simulink model "REV3"  (R2025b)
settings: Solver=ode8  StartTime=0.0  StopTime=inf  FixedStep=0.0001  RelTol=1e-3
undefined symbols (not defined in the file): BMS_Contactor_Command, MC_DC_State, MC_VSM_State, UC_State
(part 2 of 2)

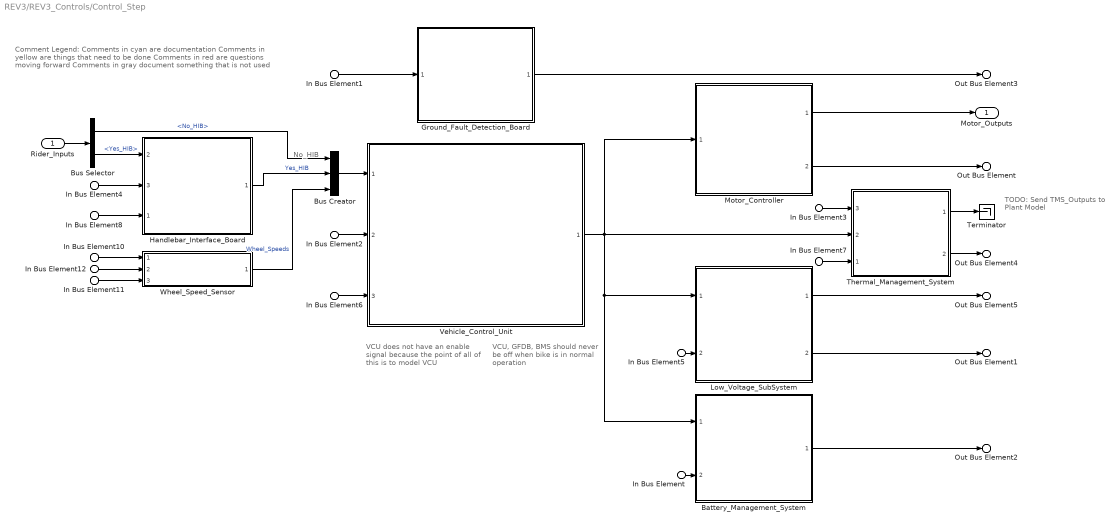
== system REV3/REV3_Controls/Control_Step ==
  note: VCU does not have an enable signal because the point of all of this is to model VCU
  note: No_HIB
  note: TODO: Send TMS_Outputs to Plant Model
  note: VCU, GFDB, BMS should never be off when bike is in normal operation
  note: Comment Legend:
      | Comments in cyan are documentation
      | Comments in yellow are things that need to be done
      | Comments in red are questions moving forward
      | Comments in gray document something that is not used
  Rider_Inputs : Inport
  In Bus Element2 : Inport  Port=2  PortName=Fault_Inputs  Element=VCU
  In Bus Element3 : Inport  Port=2  PortName=Fault_Inputs  Element=TMS
  In Bus Element4 : Inport  Port=2  PortName=Fault_Inputs  Element=HIB
  In Bus Element5 : Inport  Port=2  PortName=Fault_Inputs  Element=LVSS
  In Bus Element : Inport  Port=2  PortName=Fault_Inputs  Element=BMS
  In Bus Element1 : Inport  Port=2  PortName=Fault_Inputs  Element=GFDB
  In Bus Element12 : Inport  Port=2  PortName=Fault_Inputs  Element=WSS
  In Bus Element11 : Inport  Port=3  PortName=Sensor_Inputs
  In Bus Element6 : Inport  Port=4  PortName=Feedback_Input
  In Bus Element8 : Inport  Port=4  PortName=Feedback_Input  Element=LVSS_Outputs.HIB_Power
  In Bus Element7 : Inport  Port=4  PortName=Feedback_Input  Element=LVSS_Outputs.TMS_Power
  In Bus Element10 : Inport  Port=4  PortName=Feedback_Input  Element=LVSS_Outputs.Acc_Power
  Battery_Management_System : Subsystem  ReferencedSubsystem=BMS
  Bus Creator : BusCreator  Inputs=3
  Bus Selector : BusSelector  OutputSignals=No_HIB,Yes_HIB
  Ground_Fault_Detection_Board : Subsystem  ReferencedSubsystem=GFDB
  Handlebar_Interface_Board : Subsystem  ReferencedSubsystem=HIB
      settings: PortSchema="{\"entries\":[{\"content\":{\"sides\":[{\"content\":{\"connectorIds\":[\"In2\",\"In3\",\"In1\"]},\"type\":\"ConnectorPlacement.EquallySpacedRectSide\",\"uuid\":\"d395316e-44ff-49bc-a3f7-6228132a0ed7\"},{\"content\":{\"connectorIds\":[\"Out1\"],\"side\":\"RIGHT\"},\"type\":\"ConnectorPlacement.EquallySpacedRectSide\",\"uuid\":\"ce9decb3-eafb-4b20-852e-70e12e041567\"},{\"content\":{\"side\":\"TOP\"},\"type\":\"ConnectorPlacement.EquallySpacedRectSide\",\"uuid\":\"98cfcf48-4ed7-47ff-906e-b765ee02873c\"}]},\"type\":\"ConnectorPlacement.EquallySpacedConnector\",\"uuid\":\"acd5bdbc-8e2b-4710-a1b8-032d71c02eea\"}],\"packageUris\":[\"http://schema.mathworks.com/mf0/Connector/R2020b\"],\"version\":\"1.0\"}"
  Low_Voltage_SubSystem : Subsystem  ReferencedSubsystem=LVSS
  Motor_Controller : Subsystem  ReferencedSubsystem=PM100DXR_MC
  Terminator : Terminator
  Thermal_Management_System : Subsystem  ReferencedSubsystem=TMS
      settings: PortSchema="{\"entries\":[{\"content\":{\"sides\":[{\"content\":{\"connectorIds\":[\"In3\",\"In2\",\"In1\"]},\"type\":\"ConnectorPlacement.EquallySpacedRectSide\",\"uuid\":\"dd8c9be4-6385-48f4-820c-21f57a7ceb56\"},{\"content\":{\"connectorIds\":[\"Out1\",\"Out2\"],\"side\":\"RIGHT\"},\"type\":\"ConnectorPlacement.EquallySpacedRectSide\",\"uuid\":\"085fe805-ddf2-4eb6-90d1-73724368fca3\"},{\"content\":{\"side\":\"TOP\"},\"type\":\"ConnectorPlacement.EquallySpacedRectSide\",\"uuid\":\"ee1be840-9c3d-4e36-b4d8-a6a5862bddde\"}]},\"type\":\"ConnectorPlacement.EquallySpacedConnector\",\"uuid\":\"65698d28-aa3b-4376-ad91-6c8d073967cf\"}],\"packageUris\":[\"http://schema.mathworks.com/mf0/Connector/R2020b\"],\"version\":\"1.0\"}"
  Vehicle_Control_Unit : Subsystem  ReferencedSubsystem=VCU
  Wheel_Speed_Sensor : Subsystem  ReferencedSubsystem=WSS
  Motor_Outputs : Outport
  Out Bus Element : Outport  Port=2  PortName=Feedback_Output  Element=MC_Feedback
  Out Bus Element1 : Outport  Port=2  PortName=Feedback_Output  Element=LVSS_Feedback
  Out Bus Element2 : Outport  Port=2  PortName=Feedback_Output  Element=BMS_Feedback
  Out Bus Element4 : Outport  Port=2  PortName=Feedback_Output  Element=TMS_Feedback
  Out Bus Element5 : Outport  Port=2  PortName=Feedback_Output  Element=LVSS_Outputs
  Out Bus Element3 : Outport  Port=2  PortName=Feedback_Output  Element=GFDB_Feedback
  wires:
  Vehicle_Control_Unit/1 -> Battery_Management_System/1, Low_Voltage_SubSystem/1, Thermal_Management_System/2, Motor_Controller/1
  Motor_Controller/2 -> Out Bus Element/1
  Motor_Controller/1 -> Motor_Outputs/1
  In Bus Element6/1 -> Vehicle_Control_Unit/3
  Battery_Management_System/1 -> Out Bus Element2/1
  In Bus Element2/1 -> Vehicle_Control_Unit/2
  Thermal_Management_System/1 -> Terminator/1
  Thermal_Management_System/2 -> Out Bus Element4/1
  Bus Creator/1 -> Vehicle_Control_Unit/1
  Handlebar_Interface_Board/1 -> Bus Creator/2  "Yes_HIB"
  Rider_Inputs/1 -> Bus Selector/1
  Bus Selector/1 -> Bus Creator/1  "<No_HIB>"
  In Bus Element5/1 -> Low_Voltage_SubSystem/2
  Low_Voltage_SubSystem/2 -> Out Bus Element1/1
  In Bus Element/1 -> Battery_Management_System/2
  In Bus Element4/1 -> Handlebar_Interface_Board/3
  Bus Selector/2 -> Handlebar_Interface_Board/2  "<Yes_HIB>"
  In Bus Element3/1 -> Thermal_Management_System/3
  Low_Voltage_SubSystem/1 -> Out Bus Element5/1
  In Bus Element7/1 -> Thermal_Management_System/1
  In Bus Element8/1 -> Handlebar_Interface_Board/1
  In Bus Element1/1 -> Ground_Fault_Detection_Board/1
  Ground_Fault_Detection_Board/1 -> Out Bus Element3/1
  In Bus Element12/1 -> Wheel_Speed_Sensor/2
  In Bus Element11/1 -> Wheel_Speed_Sensor/3
  In Bus Element10/1 -> Wheel_Speed_Sensor/1
  Wheel_Speed_Sensor/1 -> Bus Creator/3  "Wheel_Speeds"

== system REV3/Plant_Model/Wheel_Speed/Aerodynamic Drag Force ==
  Speed : Inport
  Air Density : Constant  Value=1.25
  Drag Coeeficient : Gain  Gain=0.68
  Frontal Area : Gain  Gain=0.68
  Multiply : Gain  Gain=0.5
  Product : Product
  Square : Math  Operator=square
  Fad : Outport
  wires:
  Multiply/1 -> Frontal Area/1
  Frontal Area/1 -> Drag Coeeficient/1
  Air Density/1 -> Multiply/1
  Speed/1 -> Square/1
  Drag Coeeficient/1 -> Product/1
  Square/1 -> Product/2
  Product/1 -> Fad/1

== system REV3/Plant_Model/Wheel_Speed/Gradient Force ==
  Gravitational Constant : Gain  Gain=9.8
  Inclination Angle : Constant  Value=0
  Mass : Gain  Gain=200
  Sin : Trigonometry
  Fhc : Outport
  wires:
  Inclination Angle/1 -> Sin/1
  Sin/1 -> Mass/1
  Mass/1 -> Gravitational Constant/1
  Gravitational Constant/1 -> Fhc/1

== system REV3/Plant_Model/Wheel_Speed/Rolling Resistance ==
  Constant : Constant  Value=0.015
  Gravitational Constant : Gain  Gain=9.8
  Mass : Gain  Gain=200
  Frr : Outport
  wires:
  Constant/1 -> Mass/1
  Mass/1 -> Gravitational Constant/1
  Gravitational Constant/1 -> Frr/1
